simulink library "els"  (R2018b)
settings: Solver=VariableStepAuto  StartTime=0.0  StopTime=10.0  RelTol=1e-3
settings Model: Creator=dengzhe  LastModifiedBy=dengzhe
settings SFSimCC: SimUserSources=on_event.c  SimUserLibraries=libels.a  SimUseLocalCustomCode=off  SimParseCustomCode=off
settings SFSimCC: SimCustomHeaderCode=|
  | #include "els_svm.h"
  | #include "els_pid.h"
  | #include "els_pll.h"
  | #include "els_utility.h"

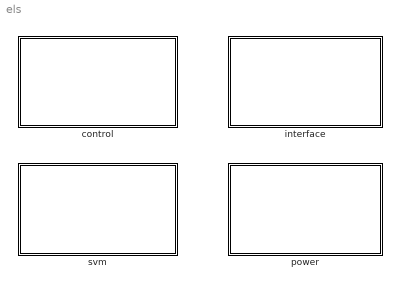
== system els ==
  control : Subsystem
  interface : Subsystem
  power : Subsystem
  svm : Subsystem

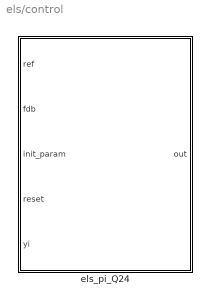
== system els/control ==
  els_pi_Q24 : Stateflow chart  TreatAsAtomicUnit=on

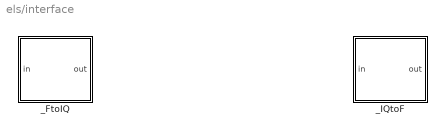
== system els/interface ==
  _FtoIQ : Stateflow chart  TreatAsAtomicUnit=on  mask{frac_num=18}
  _IQtoF : Stateflow chart  TreatAsAtomicUnit=on  mask{frac_num=18}

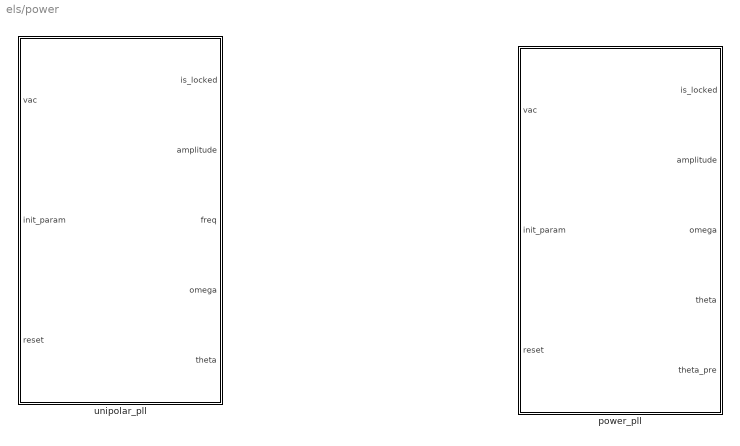
== system els/power ==
  power_pll : Stateflow chart  TreatAsAtomicUnit=on
  unipolar_pll : Stateflow chart  TreatAsAtomicUnit=on

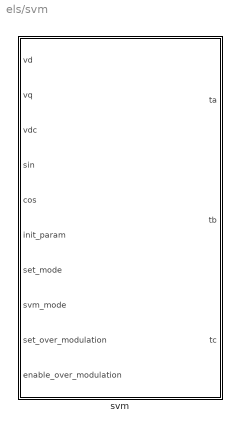
== system els/svm ==
  svm : Stateflow chart  TreatAsAtomicUnit=on

== stateflow chart els/control/els_pi_Q24 ==
  state update
    during:
    self.ref = ref;
    self.fdb = fdb;
    els_pi_update_Q24(&self);
    out = self.out;
  (default) -> (junction 3)
  (junction 3) -> update : {els_pi_init_Q24(&self, &init_param);}
  update -> (junction 21) : [reset]
  (junction 23) -> update
  (junction 21) -> (junction 23) : {
      | els_pi_reset_Q24(&self, yi);
      | out = self.out;
      | }
  data: ref input int32; fdb input int32; out output double; self local Bus: ElsPi_Q24; init_param input Bus: ElsPiInitParam_Q24; reset input boolean; yi input int32

== stateflow chart els/interface/_IQtoF ==
  (default) -> (junction 17)
  (junction 17) -> (junction 19) : {out = in / pow(2., frac_num);}
  (junction 19) -> (junction 21)
  data: in input; out output; frac_num parameter

== stateflow chart els/power/unipolar_pll ==
  state update
    during:
    self.vac = vac;
    els_unipolar_pll_update_1ms(&self);
    is_locked = self.is_locked;
    amplitude = self.amplitude;
    freq = self.freq;
    omega = self.omega;
    theta = self.theta;
  (default) -> (junction 3)
  (junction 3) -> update : {els_unipolar_pll_init(&self, &init_param);}
  update -> (junction 36) : [reset]
  (junction 38) -> update
  (junction 36) -> (junction 38) : {els_unipolar_pll_reset(&self);}
  data: vac input int32; self local Bus: ElsUnipolarPll; init_param input Bus: ElsUnipolarPllInitParam; is_locked output boolean; amplitude output int32; freq output int32; omega output int32; theta output int32; reset input

== stateflow chart els/interface/_FtoIQ ==
  (default) -> (junction 17)
  (junction 17) -> (junction 19) : {out = in * pow(2, frac_num);}
  (junction 19) -> (junction 21)
  data: in input; out output int32; frac_num parameter

== stateflow chart els/svm/svm ==
  state update
    during:
    self.vd = vd;
    self.vq = vq;
    self.vdc = vdc;
    self.sin = sin;
    self.cos = cos;
    els_svm_update(&self);
    ta = self.ta;
    tb = self.tb;
    tc = self.tc;
  (default) -> (junction 3)
  (junction 3) -> update : {els_svm_init(&self, &init_param);}
  update -> (junction 36) [order 2] : [set_mode]
  (junction 38) -> update
  update -> (junction 44) [order 1] : [set_over_modulation]
  (junction 36) -> (junction 38) : {els_svm_set_mode(&self, svm_mode);}
  (junction 44) -> (junction 38) : {els_svm_enable_over_modulation(&self, enable_over_modulation);}
  data: vd input; vq input; vdc input; sin input; cos input; self local Bus: ElsSvm; init_param input Bus: ElsSvmInitParam; set_mode input; svm_mode input; set_over_modulation input; ta output double; tb output double; tc output double; enable_over_modulation input

== stateflow chart els/power/power_pll ==
  state update
    during:
    self.vac = vac;
    els_ppll_update(&self);
    is_locked = self.is_locked;
    amplitude = self.amplitude;
    omega = self.omega;
    theta = self.theta;
    theta_pre = self.theta_pre;
  (default) -> (junction 3)
  (junction 3) -> update : {els_ppll_init(&self, &init_param);}
  update -> (junction 36) : [reset]
  (junction 38) -> update
  (junction 36) -> (junction 38) : {els_ppll_reset(&self);}
  data: vac input int32; self local Bus: ElsPpll; init_param input Bus: ElsPpllInitParam; is_locked output boolean; amplitude output int32; omega output int32; theta output int32; theta_pre output int32; reset input boolean
